simulink model "PassCarModel_RL_config"  (R2024b)
settings: Solver=FixedStepAuto  StartTime=0.0  StopTime=Tf  FixedStep=.001  RelTol=1e-2
StartFcn:
  | %tic
StopFcn:
  | %toc
model workspace (MAT data in the model file):
  AverageTimeInterval = 0.5
  Downshift_Speeds = [9.5625  23.0625  36.5625  47.8125  59.0625  68.90625  78.75; 12.9375  26.4375  39.9375  51.1875  62.4375  72.84375  83.25; 16.3125  29.8125  43.3125  54.5625  65.8125  76.78125  87.75; 19.6875  33.1875  46.6875  57.9375  69.1875  80.71875  92.25]
  EEC_Counter = Simulink.Parameter
  EEC_Counter.Value = 0
  EEC_Counter.Complexity = 'real'
  EEC_Counter.Dimensions = [1 1]
  EEC_Counter.DataType = 'uint8'
  EngRevLim = 7000
  FuzzOffset = Simulink.Parameter
  FuzzOffset.Value = 0
  FuzzOffset.Complexity = 'real'
  FuzzOffset.Dimensions = [1 1]
  FuzzOffset.DataType = 'auto'
  FuzzRange = Simulink.Parameter
  FuzzRange.Value = 60
  FuzzRange.Complexity = 'real'
  FuzzRange.Dimensions = [1 1]
  FuzzRange.DataType = 'auto'
  Fuzzing = Simulink.Parameter
  Fuzzing.Value = 0
  Fuzzing.Complexity = 'real'
  Fuzzing.Dimensions = [1 1]
  Fuzzing.DataType = 'auto'
  Pedal_Positions = [0.1 0.4 0.5 0.9]
  TrackPoints = [0 36.336 72.672 109.008 145.344 181.68 218.016 254.352 290.688 327.024 363.36 403.196036522 ... (360 elements, 120x3)]
  Upshift_Speeds = [12.9375  26.4375  39.9375  51.1875  62.4375  72.84375  83.25; 16.3125  29.8125  43.3125  54.5625  65.8125  76.78125  87.75; 19.6875  33.1875  46.6875  57.9375  69.1875  80.71875  92.25; 33  52.5  77.25  100.5  138.75  161.875  185]
  VEH.Mass = 1181
  VEH.StaticNormalFrontLoad.FR = 264.666666667
  VEH.StaticNormalFrontLoad.FL = 264.666666667
  VEH.StaticNormalRearLoad.RR = 322
  VEH.StaticNormalRearLoad.RL = 322
  VEH.WheelBase = 3.075
  VEH.FrontAxlePositionfromCG = 1.515
  VEH.RearAxlePositionfromCG = 1.504
  VEH.HeightCG = 0.134
  VEH.FrontalArea = 2.11
  VEH.DragCoefficient = 0.33
  VEH.NumberOfWheelsPerAxle = 2
  VEH.PitchMomentInertia = 1922.66666667
  VEH.RollMomentInertia = 432.333333333
  VEH.YawMomentInertia = 2066
  VEH.SteeringRatio = 18
  VEH.TrackWidth = 1.922
  VEH.SprungMass = 1096.72266667
  VEH.InitialLongPosition = 7.25329912144
  VEH.InitialLatPosition = 1.0710379423
  VEH.InitialVertPosition = 0
  VEH.InitialRollAngle = 0
  VEH.InitialPitchAngle = 0
  VEH.InitialYawAngle = 2.62319668541
  VEH.InitialLongVel = 0
  VEH.InitialLatVel = 0
  VEH.InitialVertVel = 0
  VEH.InitialRollRate = 0
  VEH.InitialPitchRate = 0
  VEH.InitialYawRate = 0
  VEH.UnsprungMassRearAxle = 160
  VEH.UnsprungMassFrontAxle = 100
  gradbp = Simulink.Parameter
  gradbp.Value = [0 3.12151852564 6.24303705128 9.36455557691 12.4860741026 15.6075926282 18.7291111538 21.8506296795 24.9721482051 28.0936667307 31.2151852564 34.336703782 37.4582223077 40.5797408333 43.7012593589 46.8227778846 49.9442964102 53.0658149359 56.1873334615 59.3088519871 62.4303705128 65.5518890384 68.673407564 71.7949260897 74.9164446153 78.037963141 81.1594816666 84.2810001922 87.4025187179 90.5240372435 93.6455557691 96.7670742948 99.8885928204 103.010111346 106.131629872 109.253148397 112.374666923 115.496185449 118.617703974 121.7392225]
  gradbp.Complexity = 'real'
  gradbp.Dimensions = [1 40]
  gradbp.DataType = 'auto'
  origin = Simulink.Parameter
  origin.Value = [47.47664 19.05601 0]
  origin.Complexity = 'real'
  origin.Dimensions = [1 3]
  origin.DataType = 'auto'
  rayDirections = [0  0  -1; 0  0  -1; 0  0  -1; 0  0  -1; 0  0  -1; 0  0  -1; 0  0  -1; 0  0  -1; 0  0  -1; 0  0  -1; 0  0  -1; 0  0  -1; 0  0  -1; 0  0  -1; 0  0  -1; 0  0  -1; 0  0  -1; 0  0  -1; 0  0  -1; 0  0  -1; 0  0  -1; 0  0  -1; 0  0  -1; 0  0  -1; 0  0  -1; 0  0  -1; 0  0  -1; 0  0  -1; 0  0  -1; 0  0  -1; 0  0  -1; 0  0  -1; 0  0  -1; 0  0  -1; 0  0  -1; 0  0  -1; 0  0  -1; 0  0  -1; 0  0  -1; 0  0  -1; 0  0  -1; 0  0  -1; 0  0  -1; 0  0  -1; 0  0  -1; 0  0  -1; 0  0  -1; 0  0  -1; 0  0  -1; 0  0  -1; 0  0  -1; 0  0  -1; 0  0  -1; 0  0  -1; 0  0  -1; 0  0  -1; 0  0  -1; 0  0  -1; 0  0  -1; 0  0  -1; 0  0  -1; 0  0  -1; 0  0  -1; 0  0  -1; 0  0  -1; 0  0  -1; 0  0  -1; 0  0  -1; 0  0  -1; 0  0  -1; 0  0  -1; 0  0  -1; 0  0  -1; 0  0  -1; 0  0  -1; 0  0  -1; 0  0  -1; 0  0  -1; 0  0  -1; 0  0  -1; 0  0  -1; 0  0  -1; 0  0  -1; 0  0  -1; 0  0  -1; 0  0  -1; 0  0  -1; 0  0  -1; 0  0  -1; 0  0  -1; 0  0  -1; 0  0  -1; 0  0  -1; 0  0  -1; 0  0  -1; 0  0  -1; 0  0  -1; 0  0  -1; 0  0  -1; 0  0  -1; 0  0  -1; 0  0  -1; 0  0  -1; 0  0  -1; 0  0  -1; 0  0  -1; 0  0  -1; 0  0  -1; 0  0  -1; 0  0  -1; 0  0  -1; 0  0  -1; 0  0  -1; 0  0  -1; 0  0  -1; 0  0  -1; 0  0  -1; 0  0  -1; 0  0  -1; 0  0  -1; 0  0  -1]
  rayLengths = [20; 20; 20; 20; 20; 20; 20; 20; 20; 20; 20; 20; 20; 20; 20; 20; 20; 20; 20; 20; 20; 20; 20; 20; 20; 20; 20; 20; 20; 20; 20; 20; 20; 20; 20; 20; 20; 20; 20; 20; 20; 20; 20; 20; 20; 20; 20; 20; 20; 20; 20; 20; 20; 20; 20; 20; 20; 20; 20; 20; 20; 20; 20; 20; 20; 20; 20; 20; 20; 20; 20; 20; 20; 20; 20; 20; 20; 20; 20; 20; 20; 20; 20; 20; 20; 20; 20; 20; 20; 20; 20; 20; 20; 20; 20; 20; 20; 20; 20; 20; 20; 20; 20; 20; 20; 20; 20; 20; 20; 20; 20; 20; 20; 20; 20; 20; 20; 20; 20; 20; 20]
  rayOrigins = [0.5  -0.5  0; 0.4  -0.5  0; 0.3  -0.5  0; 0.2  -0.5  0; 0.1  -0.5  0; 0  -0.5  0; -0.1  -0.5  0; -0.2  -0.5  0; -0.3  -0.5  0; -0.4  -0.5  0; -0.5  -0.5  0; 0.5  -0.4  0; 0.4  -0.4  0; 0.3  -0.4  0; 0.2  -0.4  0; 0.1  -0.4  0; 0  -0.4  0; -0.1  -0.4  0; -0.2  -0.4  0; -0.3  -0.4  0; -0.4  -0.4  0; -0.5  -0.4  0; 0.5  -0.3  0; 0.4  -0.3  0; 0.3  -0.3  0; 0.2  -0.3  0; 0.1  -0.3  0; 0  -0.3  0; -0.1  -0.3  0; -0.2  -0.3  0; -0.3  -0.3  0; -0.4  -0.3  0; -0.5  -0.3  0; 0.5  -0.2  0; 0.4  -0.2  0; 0.3  -0.2  0; 0.2  -0.2  0; 0.1  -0.2  0; 0  -0.2  0; -0.1  -0.2  0; -0.2  -0.2  0; -0.3  -0.2  0; -0.4  -0.2  0; -0.5  -0.2  0; 0.5  -0.1  0; 0.4  -0.1  0; 0.3  -0.1  0; 0.2  -0.1  0; 0.1  -0.1  0; 0  -0.1  0; -0.1  -0.1  0; -0.2  -0.1  0; -0.3  -0.1  0; -0.4  -0.1  0; -0.5  -0.1  0; 0.5  0  0; 0.4  0  0; 0.3  0  0; 0.2  0  0; 0.1  0  0; 0  0  0; -0.1  0  0; -0.2  0  0; -0.3  0  0; -0.4  0  0; -0.5  0  0; 0.5  0.1  0; 0.4  0.1  0; 0.3  0.1  0; 0.2  0.1  0; 0.1  0.1  0; 0  0.1  0; -0.1  0.1  0; -0.2  0.1  0; -0.3  0.1  0; -0.4  0.1  0; -0.5  0.1  0; 0.5  0.2  0; 0.4  0.2  0; 0.3  0.2  0; 0.2  0.2  0; 0.1  0.2  0; 0  0.2  0; -0.1  0.2  0; -0.2  0.2  0; -0.3  0.2  0; -0.4  0.2  0; -0.5  0.2  0; 0.5  0.3  0; 0.4  0.3  0; 0.3  0.3  0; 0.2  0.3  0; 0.1  0.3  0; 0  0.3  0; -0.1  0.3  0; -0.2  0.3  0; -0.3  0.3  0; -0.4  0.3  0; -0.5  0.3  0; 0.5  0.4  0; 0.4  0.4  0; 0.3  0.4  0; 0.2  0.4  0; 0.1  0.4  0; 0  0.4  0; -0.1  0.4  0; -0.2  0.4  0; -0.3  0.4  0; -0.4  0.4  0; -0.5  0.4  0; 0.5  0.5  0; 0.4  0.5  0; 0.3  0.5  0; 0.2  0.5  0; 0.1  0.5  0; 0  0.5  0; -0.1  0.5  0; -0.2  0.5  0; -0.3  0.5  0; -0.4  0.5  0; -0.5  0.5  0]
  theta = Simulink.Parameter
  theta.Value = [0.635451508064; 0.635451508064; 0.635451508064; 0.635451508064; 0.635451508064; 0.635451508064; 0.635451508064; 0.624762119358; 0.623142229392; 0.621522339426; 0.619902449459; 0.618282559493; 0.616662669527; 0.615042779561; 0.613422889595; 0.611802999629; 0.611153158573; 0.611153158573; 0.611153158573; 0.611153158573; 0.611153158573; 0.611153158573; 0.611153158573; 0.611153158573; 0.611278748463; 0.622335874545; 0.621279829225; 0.620168434025; 0.619057038825; 0.617945643626; 0.616834248426; 0.615722853226; 0.614611458026; 0.595312478773; 0.594482230575; 0.594482230575; 0.594482230575; 0.594482230575; 0.594482230575; 0.594482230575]
  theta.Complexity = 'real'
  theta.Dimensions = [40 1]
  theta.DataType = 'auto'
  totalDistance = Simulink.Parameter
  totalDistance.Value = 121.7392225
  totalDistance.Complexity = 'real'
  totalDistance.Dimensions = [1 1]
  totalDistance.DataType = 'auto'
  vel_profile3 = Simulink.Parameter
  vel_profile3.Value = [1; 4.4417464081; 5.58369016682; 7.3294091164; 8.57061065054; 9.62904493054; 10.5728796274; 11.4345982514; 12.2332634698; 12.981352122; 13.6876153753; 14.358495835; 14.9989108849; 15.5865267169; 16.0408872489; 16.3678958423; 16.5727345417; 16.66; 16.66; 16.66; 16.66; 16.66; 16.66; 16.66; 16.66; 16.66; 16.66; 16.66; 16.66; 16.66; 16.66; 16.66; 16.66; 16.66; 16.66; 15.8266070222; 12.4946070222; 9.16260702218; 0; 0]
  vel_profile3.Complexity = 'real'
  vel_profile3.Dimensions = [40 1]
  vel_profile3.DataType = 'auto'
  xEast = Simulink.Parameter
  xEast.Value = [0; 2.51220993996; 5.02441987992; 7.53662981988; 10.0488397598; 12.5610496998; 15.0732596398; 17.5854695797; 20.0976795197; 22.6364013732; 25.1928840476; 27.7493667221; 30.3058493965; 32.862332071; 35.4188147455; 37.9752974199; 40.5317800944; 43.0882627688; 45.6447454433; 48.2012281178; 50.7577107922; 53.3141934667; 55.8706761411; 58.4271588156; 60.9836414901; 63.5401241645; 66.096606839; 68.6530895134; 71.2095721879; 73.7660548624; 76.3225375368; 78.8790202113; 81.4317288843; 83.6574125711; 86.2417511267; 88.8277375705; 91.4137240144; 93.9997104582; 96.5856969021; 99.1716833459]
  xEast.Complexity = 'real'
  xEast.Dimensions = [40 1]
  xEast.DataType = 'auto'
  yNorth = Simulink.Parameter
  yNorth.Value = [0; 1.85274907191; 3.70549814382; 5.55824721574; 7.41099628765; 9.26374535956; 11.1164944315; 12.9692435034; 14.8219925753; 16.6378635224; 18.429029132; 20.2201947417; 22.0113603513; 23.8025259609; 25.5936915705; 27.3848571802; 29.1760227898; 30.9671883994; 32.758354009; 34.5495196186; 36.3406852283; 38.1318508379; 39.9230164475; 41.7141820571; 43.5053476667; 45.2965132764; 47.087678886; 48.8788444956; 50.6700101052; 52.4611757148; 54.2523413245; 56.0435069341; 57.8392073973; 60.0278622426; 61.7781760106; 63.5264757613; 65.2747755119; 67.0230752625; 68.7713750132; 70.5196747638]
  yNorth.Complexity = 'real'
  yNorth.Dimensions = [40 1]
  yNorth.DataType = 'auto'
undefined symbols (not defined in the file or in its folder): DecelR, DiscIntNeverNeededParam, dspblkCoreblockFVToolHelper, FO_max, FO_min, FR_max, FR_min, gcbh, ODevR, Sim3dSensor, Ts
libraries: simulink x20, dspstat3 x8, autolibutils x6, sim3dgroundtruthsensorlib x2, rllib x1, slpidlib x1, autolibtranscontrolscommon x1, vehdynlibdriver x1, sharedtransform x1, vehdynlibviscommon x1, vehdynlibsens x1
(part 1 of 5)
settings Model: DataDictionary=VehicleConfig.sldd  SimulationMode=accelerator  PauseTimes=23.4  PacingRate=0.400000  Creator=The MathWorks, Inc.  LastModifiedBy=user
settings SolverCC: SolverJacobianMethodControl=FullPerturbation  ZeroCrossAlgorithm=Adaptive  AlgebraicLoopSolver=TrustRegion  AutoInsertRateTranBlk=on  InsertRTBMode=Never (minimum delay)  DecoupledContinuousIntegration=on  MinimalZcImpactIntegration=on  MaxZcPerStep=1
settings DataIOCC: DSMLogging=off
settings OptimizationCC: UseDivisionForNetSlopeComputation=on  UseFloatMulNetSlope=on  OptimizeBlockIOStorage=off  BufferReuse=off  ReuseModelBlockBuffer=off  GlobalBufferReuse=off  ExpressionFolding=off  EnableMemcpy=off  PassReuseOutputArgsAs=Individual arguments  LocalBlockOutputs=off  ZeroExternalMemoryAtStartup=off  ZeroInternalMemoryAtStartup=off  EfficientFloat2IntCast=on  OptimizeDataStoreBuffers=off  BusAssignmentInplaceUpdate=off  OptimizationLevel=level0  OptimizationCustomize=off  EfficientTunableParamExpr=on
settings DebuggingCC: ReadBeforeWriteMsg=DisableAll  WriteAfterWriteMsg=DisableAll  WriteAfterReadMsg=DisableAll  ArtificialAlgebraicLoopMsg=none  MaskedZcDiagnostic=none  IgnoredZcDiagnostic=none  InheritedTsInSrcMsg=none  MultiTaskDSMMsg=none  IntegerOverflowMsg=none  ParamPrecisionLossAbsoluteDiffThreshold=1e-06  ParameterTunabilityLossMsg=error  UnconnectedInputMsg=warning  UnconnectedOutputMsg=warning  UnconnectedLineMsg=warning  PregeneratedLibrarySubsystemCodeDiagnostic=none  ArithmeticOperatorsInVariantConditions=warning
settings HardwareCC: ProdLongLongMode=on  TargetBitPerPointer=64  TargetBitPerSizeT=64  TargetBitPerPtrDiffT=64  TargetLongLongMode=on  TargetIntDivRoundTo=Zero  TargetEndianess=LittleEndian  TargetWordSize=64  TargetHWDeviceType=MATLAB Host  ProdEqTarget=off
settings ModelReferenceCC: UpdateModelReferenceTargets=IfOutOfDate  EnableRefExpFcnMdlSchedulingChecks=on  ModelReferenceMinAlgLoopOccurrences=on  PropagateSignalLabelsOutOfModel=off
settings SFSimCC: SimUseLocalCustomCode=off  MATLABDynamicMemAlloc=off
settings RTWCC: Description=Embedded Coder (host-based shared library target)  SystemTargetFile=ert_shrlib.tlc  TemplateMakefile=ert_default_tmf  PostCodeGenCommand=packNGo(buildInfo)  RTWUseLocalCustomCode=off  GPUComputeCapability=3.5  DLArmComputeVersion=19.05
settings CodeAppCC: ForceParamTrailComments=on  IgnoreCustomStorageClasses=off  MaxIdLength=50  OperatorAnnotations=on  SimulinkDataObjDesc=on  SFDataObjDesc=on  InsertBlockDesc=on
settings STFCustomTargetCC: TargetLangStandard=C99 (ISO)  MultiwordLength=256  GenerateSampleERTMain=on  ParMdlRefBuildCompliant=on  CompOptLevelCompliant=on  CombineOutputUpdateFcns=on  ERTCustomFileBanners=on  SupportNonInlinedSFcns=off  RemoveResetFunc=on  SupportVariableSizeSignals=on  MATLABClassNameForMDSCustomization=Simulink.SoftwareTarget.ERTCustomization  ModelStepFunctionPrototypeControlCompliant=on  UseToolchainInfoCompliant=on  SystemTargetFile=ert_shrlib.tlc
settings ERTTargetCC: TargetLangStandard=C99 (ISO)  GenerateSampleERTMain=on  ConcurrentExecutionCompliant=off  SupportContinuousTime=on  SupportVariableSizeSignals=on  CPPClassGenCompliant=off  InlinedParameterPlacement=Hierarchical  ERTCustomFileTemplate=example_file_process.tlc

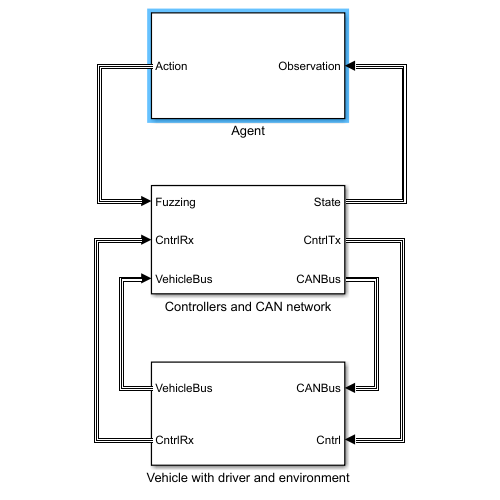
[thumbnail: Simulink's stored preview of the top-level diagram]
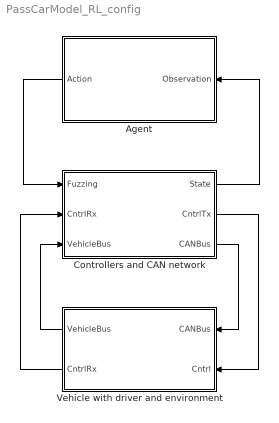
== system PassCarModel_RL_config ==
  Agent : Subsystem
  Controllers and CAN network : Subsystem
  Vehicle with driver and environment : Subsystem
  wires:
  Vehicle with driver and environment/1(VehicleBus) -> Controllers and CAN network/3(VehicleBus)
  Vehicle with driver and environment/2(CntrlRx) -> Controllers and CAN network/2(CntrlRx)
  Controllers and CAN network/2(CntrlTx) -> Vehicle with driver and environment/2(Cntrl)
  Controllers and CAN network/3(CANBus) -> Vehicle with driver and environment/1(CANBus)
  Controllers and CAN network/1(State) -> Agent/1(Observation)
  Agent/1(Action) -> Controllers and CAN network/1(Fuzzing)

== system PassCarModel_RL_config/Agent ==
  Observation : Inport
  Abs : Abs  SaturateOnIntegerOverflow=off
  Abs1 : Abs  SaturateOnIntegerOverflow=off
  Abs2 : Abs  SaturateOnIntegerOverflow=off
  Add : Sum  Inputs=+++
  Bus Selector : BusSelector  OutputSignals=AvgVehSpeed,AvgOmega
  Bus Selector1 : BusSelector  OutputSignals=AvgDecel,AvgLatAcc,OmegaDeviation
  Bus Selector2 : BusSelector  OutputSignals=AvgVehSpeed
  DecelR : Gain  Gain=DecelR
  Gain : Gain  Gain=-Ts/0.1
  Mux : Mux  Inputs=2
  ODevR : Gain  Gain=ODevR
  Policy : Subsystem
  RL Agent : rllib/RL Agent  Agent=agent  ExternalActionAsInput=off  ProvideLastAction=off  ProvideCumRwd=off  TreatAsDirectFeedthrough=on  UseStrictObservationDataTypes=off
  Relational Operator : RelationalOperator  Operator=<=  OutDataTypeStr=boolean  RndMeth=Simplest  InputSameDT=off
  StoppingCondition : Constant  Value=0.1
  Action : Outport
  wires:
  Relational Operator/1 -> RL Agent/3
  Gain/1 -> RL Agent/2  "Reward"
  Bus Selector1/3 -> Abs2/1  "<OmegaDeviation>"
  Bus Selector1/1 -> Abs/1  "<AvgDecel>"
  StoppingCondition/1 -> Relational Operator/2
  Abs1/1 -> Add/2
  RL Agent/1 -> Policy/1(action)
  Bus Selector1/2 -> Abs1/1  "<AvgLatAcc>"
  Bus Selector/1 -> Mux/1  "<AvgVehSpeed>"
  Abs/1 -> DecelR/1
  Observation/1 -> Bus Selector2/1, Bus Selector/1, Bus Selector1/1
  Add/1 -> Gain/1
  Mux/1 -> RL Agent/1  "Observation"
  Bus Selector2/1 -> Relational Operator/1  "<AvgVehSpeed>"
  Bus Selector/2 -> Mux/2  "<AvgOmega>"
  Policy/1(Action) -> Action/1  "FuzzingAction"
  Abs2/1 -> ODevR/1
  DecelR/1 -> Add/1
  ODevR/1 -> Add/3

== system PassCarModel_RL_config/Controllers and CAN network ==
  Fuzzing : Inport
  CntrlRx : Inport  Port=2
  VehicleBus : Inport  Port=3
  CAN : Subsystem
  Controllers : Subsystem
      mask Display: image('SystemControllers.png')
  Gateway : Subsystem
  Monitoring : Subsystem
  State : Outport
  CntrlTx : Outport  Port=2
  CANBus : Outport  Port=3
  wires:
  Gateway/1(OmegaFuzz) -> Monitoring/2(OmegaFuzz)
  VehicleBus/1 -> CAN/1(VehFdbk), Gateway/1(VehicleBus), Monitoring/1(VehicleBus)
  Gateway/2(CANBusOut) -> Monitoring/3(CANBus), CANBus/1, Controllers/1(CANBus)  "CANBus"
  CAN/1(CANBus) -> Gateway/2(CANBusIn)
  CntrlRx/1 -> Controllers/2(CntrlRx)
  Fuzzing/1 -> CAN/2(Fuzzing)
  Controllers/1(CntrlTx) -> CntrlTx/1
  Monitoring/1(State) -> State/1  "RLState"

== system PassCarModel_RL_config/Vehicle with driver and environment ==
  CANBus : Inport
  Cntrl : Inport  Port=2
  Driver : Subsystem
  Environment : Subsystem
      mask Display: disp('Environment')
  Passenger Vehicle : Subsystem
      mask Display: image('PassengerVehicle.png')
  Sensors : Subsystem
      mask Display: image('sensorimu.png'); % Use "Edit Image" on toolstrip to change.
  VehicleBus : Outport
  CntrlRx : Outport  Port=2
  wires:
  Environment/1(Env) -> Passenger Vehicle/4(Env), Sensors/2(Env)
  Sensors/1(CntrlRx) -> CntrlRx/1
  Passenger Vehicle/1(VehFdbk) -> Driver/1(In1), VehicleBus/1, Environment/1(VehFdbk), Sensors/1(VehFdbk)  "VehicleBus"
  Driver/1(Out1) -> Passenger Vehicle/1(Driver)
  Cntrl/1 -> Passenger Vehicle/2(Cntrl)
  CANBus/1 -> Passenger Vehicle/3(CANBus)

== system PassCarModel_RL_config/Agent/Policy ==
  action : Inport
  Bus Creator : BusCreator  Inputs=4
  Constant : Constant  Value=(FO_max+FO_min)/2
  Constant1 : Constant  Value=(FO_max-FO_min)/2
  Constant2 : Constant  Value=(FR_max+FR_min)/2
  Constant3 : Constant  Value=(FR_max-FR_min)/2
  Demux : Demux  Outputs=2
  Fuzzing : Constant
  MATLAB Function : MATLAB Function  TreatAsAtomicUnit=on
  Product : Product
  Product1 : Product
  Sum : Sum  Inputs=|++
  Sum1 : Sum  Inputs=|++
  UniformNormal : Constant  Value=0
  Action : Outport
  wires:
  Bus Creator/1 -> Action/1  "Action"
  Sum1/1 -> Bus Creator/4  "FuzzingRange"
  Fuzzing/1 -> Bus Creator/1  "Fuzzing"
  UniformNormal/1 -> Bus Creator/2  "UniformNormal"
  Sum/1 -> Bus Creator/3  "FuzzingOffset"
  Demux/1 -> Product/2
  Constant1/1 -> Product/1
  Constant/1 -> Sum/2
  Product/1 -> Sum/1
  Product1/1 -> Sum1/1
  Constant2/1 -> Sum1/2
  Constant3/1 -> Product1/1
  Demux/2 -> Product1/2
  action/1 -> MATLAB Function/1(u)
  MATLAB Function/1(y) -> Demux/1

== system PassCarModel_RL_config/Controllers and CAN network/CAN ==
  VehFdbk : Inport
  Fuzzing : Inport  Port=2
  BrakeController : Subsystem
  Bus Creator : BusCreator  Inputs=4
  CentralController : Subsystem
  EngineController : Subsystem
  TransmissionController : Subsystem
  CANBus : Outport
  wires:
  VehFdbk/1 -> TransmissionController/1(VehDataBus), CentralController/1(VehDataBus), BrakeController/2(VehDataBus), EngineController/1(VehDataBus)  "VehDataBus"
  BrakeController/1(BrakeController) -> Bus Creator/1  "BrakeController"
  EngineController/1(EngineController) -> Bus Creator/2  "EngineController"
  TransmissionController/1(TransmissionController) -> Bus Creator/3  "TransmissionController"
  CentralController/1(CentralController) -> Bus Creator/4  "CentralController"
  Bus Creator/1 -> CANBus/1
  Fuzzing/1 -> BrakeController/1(Fuzzing)

== system PassCarModel_RL_config/Controllers and CAN network/Controllers ==
  CANBus : Inport
  CntrlRx : Inport  Port=2
  ADCMode : Subsystem
  Active Differential Control : Subsystem  Variant=on  VariantControlMode=label  LabelModeActiveChoice=0
  BCMode : Subsystem  mask{ControlMode=CAN}
      mask prompts: ControlMode "Select control mode"
      mask DialogControl DescTextVar Prompt: If CAN is selected the control signals are received from the CAN bus.
  Brake Pressure Control : Subsystem  Variant=on  VariantControlMode=label  LabelModeActiveChoice=Slip control
  Bus Creator : BusCreator  Inputs=1
  Bus Creator1 : BusCreator  Inputs=1
  Bus Creator2 : BusCreator  Inputs=3
  Bus Creator3 : BusCreator  Inputs=4
  Bus Creator4 : BusCreator  Inputs=1
  ECMode : Subsystem  mask{ControlMode=CAN}
      mask prompts: ControlMode "Select control mode"
      mask DialogControl DescTextVar Prompt: If CAN is selected the control signals are received from the CAN bus.
  ECU : Subsystem  SystemSampleTime=.01
  Ground : Ground
  Logical Operator : Logic  Operator=OR  Inputs=1  AllPortsSameDT=off  OutDataTypeStr=boolean
  TCMode : Subsystem  mask{ControlMode=CAN}
      mask prompts: ControlMode "Select control mode"
      mask DialogControl DescTextVar Prompt: If CAN is selected the control signals are received from the CAN bus.
  Terminator : Terminator
  Transmission Controller : Subsystem  Variant=on  VariantControlMode=label  VariantControl=Variant1  LabelModeActiveChoice=3
  CntrlTx : Outport  VectorParamsAs1DForOutWhenUnconnected=off
  wires:
  Bus Creator/1 -> Bus Creator3/1  "ECU"
  Bus Creator1/1 -> Bus Creator3/2  "Transmission"
  Bus Creator3/1 -> CntrlTx/1  "CntrlTx"
  Bus Creator4/1 -> Bus Creator3/4  "Diff"
  Active Differential Control/1(DiffPrsCmd) -> Bus Creator4/1  "DiffPrsCmd"
  Active Differential Control/2(TrqCmd) -> [DiffTrqCmd]
  ECU/1(EngTrqCmd) -> Bus Creator/1  "EngTrqCmd"
  Transmission Controller/1(" Gear") -> Bus Creator1/1  "GearCmd"
  [DiffTrqCmd] -> ECU/1(DiffTrqCmd)  "DiffTrqCmd"
  Ground/1 -> Transmission Controller/7(UpReq), Transmission Controller/8(DownReq)
  Brake Pressure Control/2(BrkPrsCmd) -> Bus Creator2/2  "BrkPrsCmd"
  Bus Creator2/1 -> Bus Creator3/3  "Brake"
  Brake Pressure Control/1(ABSFlag) -> [ABSFlag], Logical Operator/1, Bus Creator2/1  "ABSFlag"
  ECMode/3(<ABSFlag>) -> ECU/4(ABSFlag)
  Brake Pressure Control/3(TCSFlag) -> Bus Creator2/3  "TCSFlag"
  TCMode/1(<AccFdbk>) -> Transmission Controller/1(Accel)
  TCMode/2(<DecelFdbk>) -> Transmission Controller/2(BrkCmd)
  TCMode/3(<GearFdbk>) -> Transmission Controller/3(GearReq)
  TCMode/4(<EngSpd>) -> Transmission Controller/4(EngSpd)
  TCMode/5(<Omega>) -> Transmission Controller/5(Omega)
  BCMode/1(<DecelFdbk>) -> Brake Pressure Control/1(DecelFdbk)
  BCMode/2(<Omega>) -> Brake Pressure Control/2(Omega)
  BCMode/3(Accel) -> Brake Pressure Control/3(Accel)
  BCMode/4(<AccFdbk>) -> Brake Pressure Control/4(AccelFdbk)
  BCMode/5(<BrkPrs>) -> Brake Pressure Control/5(BrkPrs)
  [ABSFlag] -> ECMode/3(ABSFlag)
  ECMode/1(<AccFdbk>) -> ECU/2(<Accel>)
  ECMode/2(<EngSpd>) -> ECU/3(EngSpd)
  [ABSFlag] -> TCMode/3(ABSFlag)
  TCMode/6(<ABSFlag>) -> Transmission Controller/6(ABSFlag)
  ADCMode/1(<AccFdbk>) -> Active Differential Control/1(Accel)
  ADCMode/2(<DecelFdbk>) -> Active Differential Control/2(BrkCmd)
  ADCMode/3(<SteerFdbk>) -> Active Differential Control/3(Steer)
  ADCMode/4(<GearFdbk>) -> Active Differential Control/4(GearFdbk)
  ADCMode/5(<Omega>) -> Active Differential Control/5(Omega)
  ADCMode/6(<Acc>) -> Active Differential Control/6(axayaz)
  ADCMode/7(<pqr>) -> Active Differential Control/7(pqr)
  Logical Operator/1 -> Terminator/1  "ABS_active"
  CANBus/1 -> BCMode/2(CANBus), TCMode/2(CANBus), ECMode/2(CANBus)
  CntrlRx/1 -> ECMode/1(CntrlRx), TCMode/1(CntrlRx), BCMode/1(CntrlRx), ADCMode/1(In1)

== system PassCarModel_RL_config/Controllers and CAN network/Gateway ==
  VehicleBus : Inport
  CANBusIn : Inport  Port=2
  BC-Filter : Subsystem
  Bus Creator : BusCreator  Inputs=4
  Bus Selector : BusSelector  OutputSignals=EngineController,BrakeController,CentralController,TransmissionController
  Terminator : Terminator
  OmegaFuzz : Outport
  CANBusOut : Outport  Port=2
  wires:
  Bus Creator/1 -> CANBusOut/1
  Bus Selector/4 -> [TC]  "<TransmissionController>"
  Bus Selector/3 -> [CC]  "<CentralController>"
  Bus Selector/2 -> Terminator/1  "<BrakeController>"
  Bus Selector/1 -> [EC]  "<EngineController>"
  CANBusIn/1 -> BC-Filter/2(CANBus), Bus Selector/1
  [EC] -> Bus Creator/1
  BC-Filter/1(BrakeController) -> Bus Creator/2  "BrakeController"
  [CC] -> Bus Creator/3
  [TC] -> Bus Creator/4
  VehicleBus/1 -> BC-Filter/1(VehicleBus)
  BC-Filter/2(OmegaFuzz) -> OmegaFuzz/1

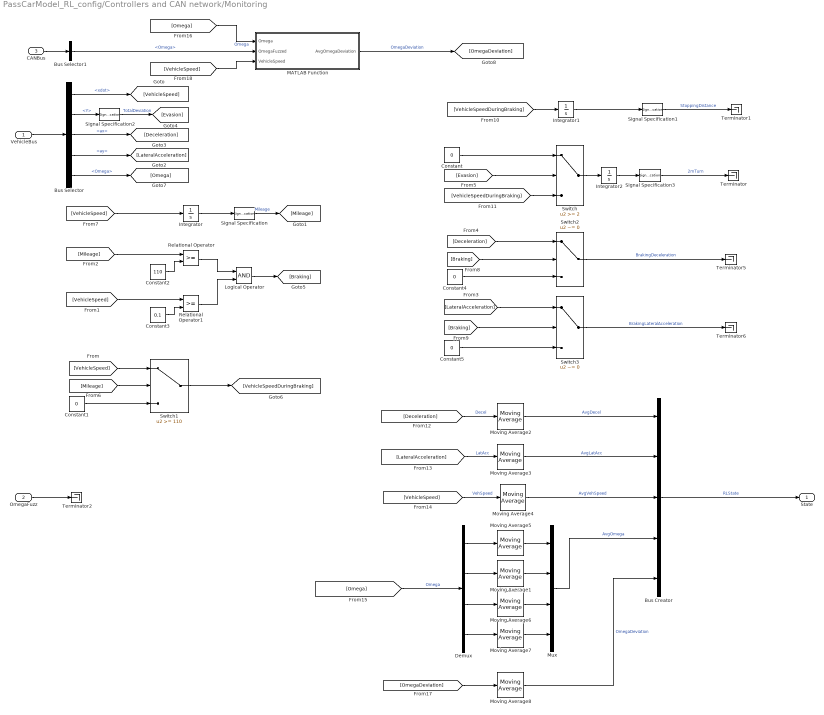
== system PassCarModel_RL_config/Controllers and CAN network/Monitoring ==
  VehicleBus : Inport
  OmegaFuzz : Inport  Port=2
  CANBus : Inport  Port=3
  Bus Creator : BusCreator  Inputs=5
  Bus Selector : BusSelector  OutputSignals=Body.BdyFrm.Cg.Vel.xdot,Body.InertFrm.Cg.Disp.Y,Body.BdyFrm.Cg.Acc.ax,Body.BdyFrm.Cg.Acc.ay,Wheels.TireFrame.Omega
  Bus Selector1 : BusSelector  OutputSignals=BrakeController.Omega
  Constant{,1,4..5} (4 alike) : Constant  Value=0
  Constant2 : Constant  Value=110
  Constant3 : Constant  Value=0.1
  Demux : Demux
  Integrator : Integrator
  Integrator1 : Integrator
  Integrator2 : Integrator
  Logical Operator : Logic  AllPortsSameDT=off  OutDataTypeStr=boolean
  MATLAB Function : MATLAB Function  TreatAsAtomicUnit=on
  Moving Average{1,5..8} (5 alike) : dspstat3/Moving Average  Method=Sliding window  ForgettingFactorPort=off  SpecifyWindowLength=on  WindowLength=50  OverlapLength=49  AllowArbitraryInputLength=off  ForgettingFactor=0.9  SimulateUsing=Code generation
  Moving Average2 : dspstat3/Moving Average  Method=Sliding window  ForgettingFactorPort=off  SpecifyWindowLength=on  WindowLength=500  OverlapLength=499  AllowArbitraryInputLength=off  ForgettingFactor=0.9  SimulateUsing=Code generation
  Moving Average3 : dspstat3/Moving Average  Method=Sliding window  ForgettingFactorPort=off  SpecifyWindowLength=on  WindowLength=500  OverlapLength=499  AllowArbitraryInputLength=off  ForgettingFactor=0.9  SimulateUsing=Code generation
  Moving Average4 : dspstat3/Moving Average  Method=Sliding window  ForgettingFactorPort=off  SpecifyWindowLength=on  WindowLength=500  OverlapLength=499  AllowArbitraryInputLength=off  ForgettingFactor=0.9  SimulateUsing=Code generation
  Mux : Mux
  Relational Operator : RelationalOperator  OutDataTypeStr=boolean  RndMeth=Simplest  InputSameDT=off
  Relational Operator1 : RelationalOperator  OutDataTypeStr=boolean  RndMeth=Simplest  InputSameDT=off
  Signal Specification{,1..3} (4 alike) : SignalSpecification  Unit=m
  Switch : Switch  Threshold=2  SaturateOnIntegerOverflow=off  InputSameDT=off
  Switch1 : Switch  Threshold=110  SaturateOnIntegerOverflow=off  InputSameDT=off
  Switch2 : Switch  Criteria=u2 ~= 0  SaturateOnIntegerOverflow=off  InputSameDT=off
  Switch3 : Switch  Criteria=u2 ~= 0  SaturateOnIntegerOverflow=off  InputSameDT=off
  Terminator{,1..2,5..6} (5 alike) : Terminator
  State : Outport
  wires:
  [VehicleSpeed] -> Switch1/1
  Integrator/1 -> Signal Specification/1
  Signal Specification/1 -> [Mileage]  "Mileage"
  VehicleBus/1 -> Bus Selector/1
  Bus Selector/2 -> Signal Specification2/1  "<Y>"
  Constant/1 -> Switch/1
  Constant1/1 -> Switch1/3
  Integrator1/1 -> Signal Specification1/1
  Switch1/1 -> [VehicleSpeedDuringBraking]
  Signal Specification1/1 -> Terminator1/1  "StoppingDistance"
  Signal Specification2/1 -> [Evasion]  "TotalDeviation"
  CANBus/1 -> Bus Selector1/1
  Switch/1 -> Integrator2/1
  Integrator2/1 -> Signal Specification3/1
  Signal Specification3/1 -> Terminator/1  "2mTurn"
  [Deceleration] -> Switch2/1
  [LateralAcceleration] -> Switch3/1
  Constant2/1 -> Relational Operator/2
  Constant3/1 -> Relational Operator1/2
  Relational Operator/1 -> Logical Operator/1
  Relational Operator1/1 -> Logical Operator/2
  Constant4/1 -> Switch2/3
  Constant5/1 -> Switch3/3
  Switch2/1 -> Terminator5/1  "BrakingDeceleration"
  Switch3/1 -> Terminator6/1  "BrakingLateralAcceleration"
  Bus Selector/1 -> [VehicleSpeed]  "<xdot>"
  [VehicleSpeed] -> Relational Operator1/1
  [Mileage] -> Relational Operator/1
  Bus Selector/4 -> [LateralAcceleration]  "<ay>"
  Bus Selector/3 -> [Deceleration]  "<ax>"
  [Evasion] -> Switch/2
  [Mileage] -> Switch1/2
  [VehicleSpeed] -> Integrator/1
  Logical Operator/1 -> [Braking]
  [Braking] -> Switch2/2
  [Braking] -> Switch3/2
  [VehicleSpeedDuringBraking] -> Integrator1/1
  [VehicleSpeedDuringBraking] -> Switch/3
  [LateralAcceleration] -> Moving Average3/1  "LatAcc"
  Bus Selector/5 -> [Omega]  "<Omega>"
  [Omega] -> Demux/1  "Omega"
  [VehicleSpeed] -> Moving Average4/1  "VehSpeed"
  [Deceleration] -> Moving Average2/1  "Decel"
  Moving Average2/1 -> Bus Creator/1  "AvgDecel"
  Moving Average3/1 -> Bus Creator/2  "AvgLatAcc"
  Moving Average4/1 -> Bus Creator/3  "AvgVehSpeed"
  Moving Average5/1 -> Mux/1
  Bus Creator/1 -> State/1  "RLState"
  Demux/1 -> Moving Average5/1
  Demux/2 -> Moving Average1/1
  Demux/3 -> Moving Average6/1
  Demux/4 -> Moving Average7/1
  Moving Average1/1 -> Mux/2
  Moving Average6/1 -> Mux/3
  Moving Average7/1 -> Mux/4
  Mux/1 -> Bus Creator/4  "AvgOmega"
  [OmegaDeviation] -> Moving Average8/1
  Bus Selector1/1 -> MATLAB Function/2(OmegaFuzzed)  "<Omega>"
  [Omega] -> MATLAB Function/1(Omega)  "Omega"
  [VehicleSpeed] -> MATLAB Function/3(VehicleSpeed)
  MATLAB Function/1(AvgOmegaDeviation) -> [OmegaDeviation]  "OmegaDeviation"
  OmegaFuzz/1 -> Terminator2/1
  Moving Average8/1 -> Bus Creator/5  "OmegaDeviation"

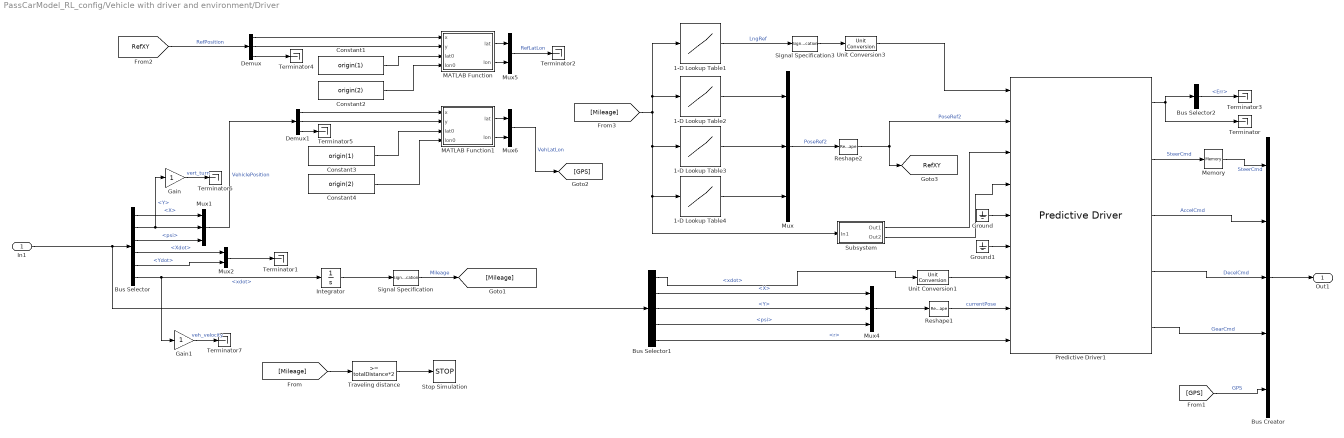
== system PassCarModel_RL_config/Vehicle with driver and environment/Driver ==
  In1 : Inport
  1-D Lookup Table1 : Lookup_n-D  NumberOfTableDimensions=1  BreakpointsForDimension1=gradbp  BeginIndexSearchUsingPreviousIndexResult=on  Table=vel_profile3  ExtrapMethod=Clip  UseLastTableValue=on  InternalRulePriority=Speed  RndMeth=Simplest
  1-D Lookup Table2 : Lookup_n-D  NumberOfTableDimensions=1  BreakpointsForDimension1=gradbp  BeginIndexSearchUsingPreviousIndexResult=on  Table=xEast  ExtrapMethod=Clip  InternalRulePriority=Speed  RndMeth=Simplest
  1-D Lookup Table3 : Lookup_n-D  NumberOfTableDimensions=1  BreakpointsForDimension1=gradbp  BeginIndexSearchUsingPreviousIndexResult=on  Table=yNorth  ExtrapMethod=Clip  InternalRulePriority=Speed  RndMeth=Simplest
  1-D Lookup Table4 : Lookup_n-D  NumberOfTableDimensions=1  BreakpointsForDimension1=gradbp  BeginIndexSearchUsingPreviousIndexResult=on  Table=theta  ExtrapMethod=Clip  InternalRulePriority=Speed  RndMeth=Simplest
  Bus Creator : BusCreator  Inputs=5
  Bus Selector : BusSelector  OutputSignals=Body.InertFrm.Cg.Disp.X,Body.InertFrm.Cg.Disp.Y,Body.InertFrm.Cg.Ang.psi,Body.InertFrm.Cg.Vel.Xdot,Body.InertFrm.Cg.Vel.Ydot,Body.BdyFrm.Cg.Vel.xdot
  Bus Selector1 : BusSelector  OutputSignals=Body.BdyFrm.Cg.Vel.xdot,Body.InertFrm.Cg.Disp.X,Body.InertFrm.Cg.Disp.Y,Body.InertFrm.Cg.Ang.psi,Body.BdyFrm.Cg.AngVel.r
  Bus Selector2 : BusSelector  OutputSignals=Err.LatErr.Err
  Constant1 : Constant  Value=origin(1)
  Constant2 : Constant  Value=origin(2)
  Constant3 : Constant  Value=origin(1)
  Constant4 : Constant  Value=origin(2)
  Demux : Demux  Outputs=3
  Demux1 : Demux  Outputs=3
  Gain : Gain
  Gain1 : Gain
  Ground : Ground
  Ground1 : Ground
  Integrator : Integrator
  MATLAB Function : MATLAB Function  TreatAsAtomicUnit=on
  MATLAB Function1 : MATLAB Function  TreatAsAtomicUnit=on
  Memory : Memory
  Mux : Mux  Inputs=3
  Mux1 : Mux  Inputs=3
  Mux2 : Mux  Inputs=2
  Mux4 : Mux  Inputs=3
  Mux5 : Mux  Inputs=2
  Mux6 : Mux  Inputs=2
  Predictive Driver1 : vehdynlibdriver/Predictive Driver  extAccelOvr=off  extDecelOvr=off  extAccelHld=off  extDecelHld=off  extAccelZero=off  extDecelZero=off  extSteerOvr=on  extSteerHld=off  extSteerZero=off  cntrlType=Predictive  cntrlTypeLat=Stanley  shftType=Reverse, Neutral, Drive  coordMode=SAE J670 (Z-down)  refType=Reference pose  velUnits=m/s  angUnits=rad  gearOut=on  steerOut=on  Kp=10  Ki=5  Kff=.1  Kg=0  VehVelVec=[0 100]  KffVec=[.1 .1]  KpVec=[10 10]  KiVec=[5 5]  KgVec=[0 0]  vnom=5  Kaw=1  tauerr=.01  tau=0.15  L=50  Kpt=15000  aR=200  bR=2.5  cR=.5  g=9.81  vecPose=on  dynamMode=on  PositionGainF=2.5  PositionGainR=2.5  YawRateGain=.2  DelayGain=.2  enableDrift=off  BetaRef=20*pi/180  KpBeta=1  KpDrift=2  KdDrift=1  KpPsi=6  KOmega=30  tOmega=1  a=VEH.FrontAxlePositionfromCG  b=VEH.RearAxlePositionfromCG  m=VEH.Mass  Cy_f=5000  Cy_r=70933  I=4013  Ksteer=18  theta=45*pi/180  Idl=3  Re=.3  lambda_mu=1  GearInit=0  tShift=.1  pdlVec=[0.1 0.4 0.5 0.9]  upShftTbl=[-1 12.9375 26.4375 39.9375 51.18749999999999 62.4375 72.84375 83.25;-1 16.3125 29.8125 43.3125 54.5624 65.8125 76.78125 87.75;-1 19.6875 33.1875 46.68749999999999 57.9375 69.1875 80.71875 92.25;-1 33 52.5 77.25 100.5 138.75 161.875 185]  dwnShftTbl=[-1 12.9375 26.4375 39.9375 51.18749999999999 62.4375 72.84375 83.25;-1 16.3125 29.8125 43.3125 54.5624 65.8125 76.78125 87.75;-1 19.6875 33.1875 46.68749999999999 57.9375 69.1875 80.71875 92.25;-1 33 52.5 77.25 100.5 138.75 161.875 185]  tClutch=.5  tRev=.5  tPark=120  UpGearVec="[0  1  2  3  4  5  6  7]"  DownGearVec="[1  2  3  4  5  6  7  8]"  aMode=2
  Reshape1 : Reshape  OutputDimensionality=Row vector (2-D)  OutputDimensions=[1,3]
  Reshape2 : Reshape  OutputDimensionality=Row vector (2-D)
  Signal Specification : SignalSpecification  Unit=m
  Signal Specification3 : SignalSpecification  Unit=m/s
  Stop Simulation : Stop
  Subsystem : Subsystem
  Terminator{,1..7} (8 alike) : Terminator
  Traveling distance : simulink/Logic and Bit Operations/Compare To Constant  relop=>=  const=totalDistance*2  OutDataTypeStr=boolean  ZeroCross=off
  Unit Conversion1 : UnitConversion
  Unit Conversion3 : UnitConversion
  Out1 : Outport
  tag scope: RefXY=global
  wires:
  Predictive Driver1/5 -> Bus Creator/4  "GearCmd"
  Bus Selector/4 -> Mux2/1  "<Xdot>"
  Predictive Driver1/1 -> Terminator/1, Bus Selector2/1
  Reshape1/1 -> Predictive Driver1/8  "currentPose"
  Ground/1 -> Predictive Driver1/5
  Predictive Driver1/2 -> Memory/1  "SteerCmd"
  Bus Selector/2 -> Mux1/2, Gain/1  "<Y>"
  Mux2/1 -> Terminator1/1
  Traveling distance/1 -> Stop Simulation/1
  Integrator/1 -> Signal Specification/1
  Bus Selector/6 -> Gain1/1, Integrator/1  "<xdot>"
  Bus Selector1/4 -> Mux4/3  "<psi>"
  Bus Selector/5 -> Mux2/2  "<Ydot>"
  Bus Creator/1 -> Out1/1
  Predictive Driver1/3 -> Bus Creator/2  "AccelCmd"
  Bus Selector1/2 -> Mux4/1  "<X>"
  Bus Selector1/1 -> Unit Conversion1/1  "<xdot>"
  Predictive Driver1/4 -> Bus Creator/3  "DecelCmd"
  Bus Selector/3 -> Mux1/3  "<psi>"
  Bus Selector/1 -> Mux1/1  "<X>"
  Bus Selector1/3 -> Mux4/2  "<Y>"
  Unit Conversion1/1 -> Predictive Driver1/7
  Signal Specification/1 -> [Mileage]  "Mileage"
  1-D Lookup Table1/1 -> Signal Specification3/1  "LngRef"
  Signal Specification3/1 -> Unit Conversion3/1
  Unit Conversion3/1 -> Predictive Driver1/1
  In1/1 -> Bus Selector/1, Bus Selector1/1
  [Mileage] -> Traveling distance/1
  [Mileage] -> Subsystem/1(In1), 1-D Lookup Table4/1, 1-D Lookup Table3/1, 1-D Lookup Table1/1, 1-D Lookup Table2/1
  [RefXY] -> Demux/1  "RefPosition"
  Mux4/1 -> Reshape1/1
  Memory/1 -> Bus Creator/1  "SteerCmd"
  1-D Lookup Table2/1 -> Mux/1
  1-D Lookup Table3/1 -> Mux/2
  1-D Lookup Table4/1 -> Mux/3
  Mux/1 -> Reshape2/1  "PoseRef2"
  Reshape2/1 -> [RefXY], Predictive Driver1/2  "PoseRef2"
  Mux1/1 -> Demux1/1  "VehiclePosition"
  MATLAB Function/1(lat) -> Mux5/1
  Demux/1 -> MATLAB Function/1(x)
  Demux/2 -> MATLAB Function/2(y)
  Constant1/1 -> MATLAB Function/3(lat0)
  Constant2/1 -> MATLAB Function/4(lon0)
  Mux5/1 -> Terminator2/1  "RefLatLon"
  MATLAB Function/2(lon) -> Mux5/2
  Demux1/1 -> MATLAB Function1/1(x)
  Demux1/2 -> MATLAB Function1/2(y)
  MATLAB Function1/2(lon) -> Mux6/2
  Mux6/1 -> [GPS]  "VehLatLon"
  MATLAB Function1/1(lat) -> Mux6/1
  Constant3/1 -> MATLAB Function1/3(lat0)
  Constant4/1 -> MATLAB Function1/4(lon0)
  Bus Selector1/5 -> Predictive Driver1/9  "<r>"
  [GPS] -> Bus Creator/5  "GPS"
  Bus Selector2/1 -> Terminator3/1  "<Err>"
  Subsystem/2(Out2) -> Predictive Driver1/4
  Subsystem/1(Out1) -> Predictive Driver1/3
  Ground1/1 -> Predictive Driver1/6
  Demux/3 -> Terminator4/1
  Demux1/3 -> Terminator5/1
  Gain/1 -> Terminator6/1  "vert_turn"
  Gain1/1 -> Terminator7/1  "veh_velocity"

== system PassCarModel_RL_config/Vehicle with driver and environment/Environment ==
  In Bus Element2 : Inport  PortName=VehFdbk
  In Bus Element8 : Inport  PortName=VehFdbk  Element=Body.InertFrm
  In Bus Element9 : Inport  PortName=VehFdbk  Element=Body.InertFrm
  In Bus Element1 : Inport  PortName=VehFdbk  Element=Body.InertFrm.Cg.Disp
  Bus Creator2 : BusCreator  Inputs=2
  Bus Selector : BusSelector  OutputSignals=FrntAxl.Lft.Disp.X,FrntAxl.Rght.Disp.X,RearAxl.Lft.Disp.X,RearAxl.Rght.Disp.X
  Bus Selector1 : BusSelector  OutputSignals=FrntAxl.Lft.Disp.Y,FrntAxl.Rght.Disp.Y,RearAxl.Lft.Disp.Y,RearAxl.Rght.Disp.Y
  Constant1 : Constant  Value=0
  Constant2 : Constant  Value=0
  Constant6 : Constant  Value=0
  Ground Feedback : Subsystem  Variant=on  VariantControlMode=label  LabelModeActiveChoice=0
  Road Track Friction : Subsystem  mask(Road Track Friction){surface_popup=Constant friction coefficient scaling factor, lambda_g=.6, lambda_r=.4, r_x0=175, r_y0=-100, r_xw=1000, r_yw=500, aMode=2}
      mask prompts: surface_popup "vdynblks:vehdynManFriction:blkPrm_surface_popup"; lambda_g "vdynblks:vehdynManFriction:blkPrm_lambda_g"; lambda_r "vdynblks:vehdynManFriction:blkPrm_lambda_r"; r_x0 "vdynblks:vehdynManFriction:blkPrm_r_x0"; r_y0 "vdynblks:vehdynManFriction:blkPrm_r_y0"; r_xw "vdynblks:vehdynManFriction:blkPrm_r_xw"; r_yw "vdynblks:vehdynManFriction:blkPrm_r_yw"
      mask init:
      | % Scaling factor for the friction coefficient around the rectangular region
      | mutable = [lambda_g, lambda_g, lambda_g, lambda_g;
      |            lambda_g, lambda_r, lambda_r, lambda_g; 
      |            lambda_g, lambda_r, lambda_r, lambda_g; 
      |            lambda_g, lambda_g, lambda_g, lambda_g ];
      |        
      | 
      | % The step is distance between breakpoint near the boundary of high and
      | % low friction coefficient
      | 
      | step = 0.01 ; 
      | 
      | % In the mask initialization, xbr and ybr breakpoints are with respect to
      | % Body fixed coordinate system. At time t=0, xbr and ybr breakpoints
      | % updates to Earth (Inertial) Fixed coordinate system. The breakpoints for
      | % the lookup table are added via inputs.
      | 
      | xbr = [(r_x0 - step) , (r_x0 + step), (r_x0 + r_xw - step) , (r_x0 + r_xw + step) ];
      | ybr = [(r_y0 - step) , (r_y0 + step), (r_y0 + r_yw - step) , (r_y0 + r_yw + step) ];
      | 
      | 
      | % To check if the created track is split mu or constant mu
      | 
      | surface_popup = get_param(gcb, 'surface_popup');
      | 
      | if strcmp(surface_popup, 'Split friction coefficient scaling factor')
      |     SplitLambdaTrck = 1;
      | elseif strcmp(surface_popup, 'Constant friction coefficient scaling factor')
      |     SplitLambdaTrck = 0;
      | end
      mask Help: eval('vdynblkshelp(''vdynblkstrack'')');
      mask TypeOptions surface_popup: vdynblks:vehdynManFriction:blkCmb_surface_popup_c1 | vdynblks:vehdynManFriction:blkCmb_surface_popup_c2
      mask Callback surface_popup:
      | surface_popup = get_param(gcb, 'surface_popup');
      | m = Simulink.Mask.get(gcb);
      | 
      | lambda_g = m.getParameter('lambda_g');
      | lambda_r = m.getParameter('lambda_r');
      | r_x0 = m.getParameter('r_x0');
      | r_y0 = m.getParameter('r_y0');
      | r_xw = m.getParameter('r_xw');
      | r_yw = m.getParameter('r_yw');
      | %track_view = m.getParameter('track_view');
      | 
      | 
      | if strcmp(surface_popup, 'Split friction coefficient scaling factor')
      |     lambda_g.Visible = 'on';
      |     lambda_r.Visible = 'on';
      |     r_x0.Visible = 'on';
      |     r_y0.Visible = 'on';
      |     r_xw.Visible = 'on';
      |     r_yw.Visible = 'on';
      |     %track_view.Visible = 'on';
      | 
      | elseif strcmp(surface_popup,'Constant friction coefficient scaling factor')
      |     lambda_g.Visible = 'on';
      |     lambda_r.Visible = 'off';
      |     r_x0.Visible = 'off';
      |     r_y0.Visible = 'off';
      |     r_xw.Visible = 'off';
      |     r_yw.Visible = 'off';
      |     %track_view.Visible = 'off';
      | end
      | [~]=autosharedicon('autolibutils',gcb,0);
      mask DialogControl DescGroupVar Prompt: Road Track Friction
      mask DialogControl DescTextVar Prompt: vdynblks:vehdynManFriction:blkDesc
      mask DialogControl surface_popup Prompt: Type of surface:
      mask DialogControl lambda_g Prompt: Scaling factor for the friction coefficient of ground, lambda_g :
      mask DialogControl lambda_r Prompt: Scaling factor for the friction coefficient of rectangular surface, lambda_r :
      mask DialogControl r_x0 Prompt: X coordinate of lower left corner of rectangular surface, r_x0 [m]:
      mask DialogControl r_y0 Prompt: Y coordinate of lower left corner of rectangular surface, r_y0 [m]:
      mask DialogControl r_xw Prompt: Rectangular surface width in X direction, r_xw [m]:
      mask DialogControl r_yw Prompt: Rectangular surface width in Y direction, r_yw [m]:
  Vector Concatenate1 : Concatenate  NumInputs=3
  Wheel Coordinates : Subsystem
  Env : Outport  VectorParamsAs1DForOutWhenUnconnected=off
  wires:
  Bus Selector1/4 -> Wheel Coordinates/8(RearAxlRghtY)  "<Y>"
  Bus Selector1/3 -> Wheel Coordinates/7(RearAxlLftY)  "<Y>"
  In Bus Element9/1 -> Bus Selector1/1
  Bus Selector1/2 -> Wheel Coordinates/6(FrntAxlRghtY)  "<Y>"
  Bus Selector1/1 -> Wheel Coordinates/5(FrntAxlLftY)  "<Y>"
  In Bus Element8/1 -> Bus Selector/1
  Constant1/1 -> Vector Concatenate1/1  "X"
  Constant6/1 -> Vector Concatenate1/3  "Z"
  Bus Creator2/1 -> Env/1
  Constant2/1 -> Vector Concatenate1/2  "Y"
  Vector Concatenate1/1 -> Bus Creator2/1  "Wind"
  Ground Feedback/1(Ground) -> Bus Creator2/2  "Gnd"
  Road Track Friction/1(FricCoeffLambda) -> Ground Feedback/1(Friction)
  Wheel Coordinates/1(XWhl) -> Road Track Friction/1(XWhl)
  Wheel Coordinates/2(YWhl) -> Road Track Friction/2(YWhl)
  Bus Selector/1 -> Wheel Coordinates/1(FrntAxlLftX)  "<X>"
  Bus Selector/2 -> Wheel Coordinates/2(FrntAxlRghtX)  "<X>"
  Bus Selector/3 -> Wheel Coordinates/3(RearAxlLftX)  "<X>"
  Bus Selector/4 -> Wheel Coordinates/4(RearAxlRghtX)  "<X>"
  In Bus Element1/1 -> Road Track Friction/3(Cg)
  In Bus Element2/1 -> Ground Feedback/2(VehFdbk)

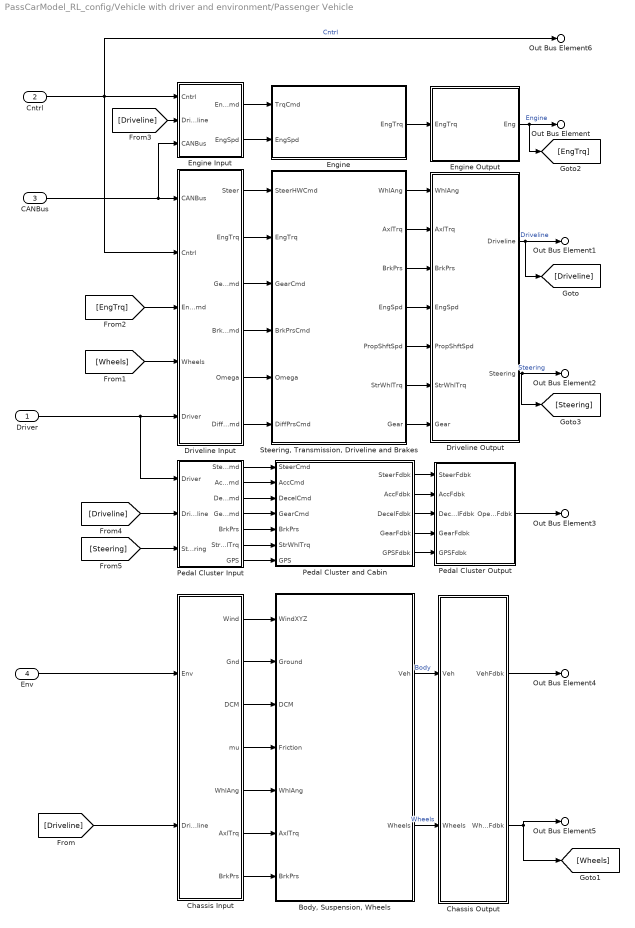
== system PassCarModel_RL_config/Vehicle with driver and environment/Passenger Vehicle ==
  Driver : Inport
  Cntrl : Inport  Port=2
  CANBus : Inport  Port=3
  Env : Inport  Port=4
  "Body, Suspension, Wheels" : Subsystem  Variant=on  VariantControlMode=label  LabelModeActiveChoice=3
  Chassis Input : Subsystem
  Chassis Output : Subsystem
  Driveline Input : Subsystem  mask{ControlMode=CAN}
      mask prompts: ControlMode "Select control mode"
      mask DialogControl DescTextVar Prompt: If CAN is selected the control signals are received from the CAN bus.
  Driveline Output : Subsystem
  Engine : Subsystem  Variant=on  VariantControlMode=label  LabelModeActiveChoice=0
  Engine Input : Subsystem  mask{ControlMode=CAN}
      mask prompts: ControlMode "Select control mode"
      mask DialogControl DescTextVar Prompt: If CAN is selected the control signals are received from the CAN bus.
  Engine Output : Subsystem
  Pedal Cluster Input : Subsystem
  Pedal Cluster Output : Subsystem
  Pedal Cluster and Cabin : Subsystem
  "Steering, Transmission, Driveline and Brakes" : Subsystem  Variant=on  VariantControlMode=label  LabelModeActiveChoice=0
  Out Bus Element : Outport  PortName=VehFdbk  Element=Engine
  Out Bus Element3 : Outport  PortName=VehFdbk  Element=Driver
  Out Bus Element4 : Outport  PortName=VehFdbk  Element=Body
  Out Bus Element5 : Outport  PortName=VehFdbk  Element=Wheels
  Out Bus Element1 : Outport  PortName=VehFdbk  Element=Driveline
  Out Bus Element2 : Outport  PortName=VehFdbk  Element=Steering
  Out Bus Element6 : Outport  PortName=VehFdbk  Element=Cntrl
  wires:
  Env/1 -> Chassis Input/1(Env)
  Chassis Input/1(Wind) -> "Body, Suspension, Wheels"/1(WindXYZ)
  "Steering, Transmission, Driveline and Brakes"/1(WhlAng) -> Driveline Output/1(WhlAng)
  "Steering, Transmission, Driveline and Brakes"/2(AxlTrq) -> Driveline Output/2(AxlTrq)
  "Steering, Transmission, Driveline and Brakes"/3(BrkPrs) -> Driveline Output/3(BrkPrs)
  "Steering, Transmission, Driveline and Brakes"/4(EngSpd) -> Driveline Output/4(EngSpd)
  "Steering, Transmission, Driveline and Brakes"/5(PropShftSpd) -> Driveline Output/5(PropShftSpd)
  Driver/1 -> Pedal Cluster Input/1(Driver), Driveline Input/5(Driver)
  Cntrl/1 -> Driveline Input/2(Cntrl), Out Bus Element6/1, Engine Input/1(Cntrl)  "Cntrl"
  Driveline Input/1(Steer) -> "Steering, Transmission, Driveline and Brakes"/1(SteerHWCmd)
  Driveline Input/3(GearCmd) -> "Steering, Transmission, Driveline and Brakes"/3(GearCmd)
  Driveline Input/4(BrkPrsCmd) -> "Steering, Transmission, Driveline and Brakes"/4(BrkPrsCmd)
  Driveline Input/5(Omega) -> "Steering, Transmission, Driveline and Brakes"/5(Omega)
  Engine/1(EngTrq) -> Engine Output/1("EngTrq ")
  Engine Input/1(EngTrqCmd) -> Engine/1(TrqCmd)
  Engine Input/2(EngSpd) -> Engine/2(EngSpd)
  Engine Output/1(Eng) -> Out Bus Element/1, [EngTrq]  "Engine"
  [Wheels] -> Driveline Input/4(Wheels)
  [EngTrq] -> Driveline Input/3(EngTrqCmd)
  [Driveline] -> Engine Input/2(Driveline)
  Driveline Input/6(DiffPrsCmd) -> "Steering, Transmission, Driveline and Brakes"/6(DiffPrsCmd)
  "Steering, Transmission, Driveline and Brakes"/6(StrWhlTrq) -> Driveline Output/6(StrWhlTrq)
  Pedal Cluster Output/1(OperatorFdbk) -> Out Bus Element3/1
  Pedal Cluster and Cabin/1(SteerFdbk) -> Pedal Cluster Output/1(SteerFdbk)
  Pedal Cluster and Cabin/2(AccFdbk) -> Pedal Cluster Output/2(AccFdbk)
  Pedal Cluster and Cabin/3(DecelFdbk) -> Pedal Cluster Output/3(DecelFdbk)
  Pedal Cluster and Cabin/4(GearFdbk) -> Pedal Cluster Output/4(GearFdbk)
  Pedal Cluster Input/4(GearCmd) -> Pedal Cluster and Cabin/4(GearCmd)
  Pedal Cluster Input/3(DecelCmd) -> Pedal Cluster and Cabin/3(DecelCmd)
  Pedal Cluster Input/2(AccelCmd) -> Pedal Cluster and Cabin/2(AccCmd)
  Pedal Cluster Input/1(SteerCmd) -> Pedal Cluster and Cabin/1(SteerCmd)
  [Driveline] -> Pedal Cluster Input/2(Driveline)
  Pedal Cluster Input/5(BrkPrs) -> Pedal Cluster and Cabin/5(BrkPrs)
  [Steering] -> Pedal Cluster Input/3(Steering)
  Pedal Cluster Input/6(StrWhlTrq) -> Pedal Cluster and Cabin/6(StrWhlTrq)
  Chassis Output/2(WheelsFdbk) -> Out Bus Element5/1, [Wheels]
  Chassis Output/1(VehFdbk) -> Out Bus Element4/1
  "Steering, Transmission, Driveline and Brakes"/7(Gear) -> Driveline Output/7(Gear)
  Driveline Output/1(Driveline) -> Out Bus Element1/1, [Driveline]  "Driveline"
  Driveline Output/2(Steering) -> [Steering], Out Bus Element2/1  "Steering"
  Chassis Input/3(DCM) -> "Body, Suspension, Wheels"/3(DCM)
  Chassis Input/6(AxlTrq) -> "Body, Suspension, Wheels"/6(AxlTrq)
  "Body, Suspension, Wheels"/1(Veh) -> Chassis Output/1(Veh)  "Body"
  "Body, Suspension, Wheels"/2(Wheels) -> Chassis Output/2(Wheels)  "Wheels"
  Chassis Input/7(BrkPrs) -> "Body, Suspension, Wheels"/7(BrkPrs)
  Chassis Input/2(Gnd) -> "Body, Suspension, Wheels"/2(Ground)
  Chassis Input/5(WhlAng) -> "Body, Suspension, Wheels"/5(WhlAng)
  Chassis Input/4(mu) -> "Body, Suspension, Wheels"/4(Friction)
  [Driveline] -> Chassis Input/2(Driveline)
  CANBus/1 -> Engine Input/3(CANBus), Driveline Input/1(CANBus)
  Driveline Input/2(EngTrq) -> "Steering, Transmission, Driveline and Brakes"/2(EngTrq)
  Pedal Cluster and Cabin/5(GPSFdbk) -> Pedal Cluster Output/5(GPSFdbk)
  Pedal Cluster Input/7(GPS) -> Pedal Cluster and Cabin/7(GPS)

== system PassCarModel_RL_config/Vehicle with driver and environment/Sensors ==
  VehFdbk : Inport
  Env : Inport  Port=2
  Bus Creator1 : BusCreator  Inputs=2
  Bus Selector : BusSelector  OutputSignals=Body.BdyFrm.Cg.Acc.ax,Body.BdyFrm.Cg.Acc.ay,Body.BdyFrm.Cg.Acc.az  OutputAsBus=on
  Bus Selector1 : BusSelector  OutputSignals=Body.BdyFrm.Cg.AngVel.p,Body.BdyFrm.Cg.AngVel.q,Body.BdyFrm.Cg.AngVel.r  OutputAsBus=on
  Bus Selector2 : BusSelector  OutputSignals=Body.BdyFrm.Cg.AngAcc.pdot,Body.BdyFrm.Cg.AngAcc.qdot,Body.BdyFrm.Cg.AngAcc.rdot  OutputAsBus=on
  Bus Selector3 : BusSelector  OutputSignals=Driver  OutputAsBus=on
  Bus Selector4 : BusSelector  OutputSignals=Engine.EngTrq,Driveline.EngSpd  OutputAsBus=on
  Bus Selector5 : BusSelector  OutputSignals=Driveline.BrkPrs,Wheels.TireFrame.Kappa,Wheels.TireFrame.Alpha,Wheels.TireFrame.Omega  OutputAsBus=on
  Bus Selector6 : BusSelector  OutputSignals=Driveline.PropShftSpd,Driveline.AxlTrq  OutputAsBus=on
  Bus to Vector : BusToVector
  Bus to Vector1 : BusToVector
  Bus to Vector2 : BusToVector
  Constant : Constant  Value=[0,0,0]
  Constant1 : Constant  Value=[0,0,9.81]
  Three-axis Inertial Measurement Unit : vehdynlibsens/Three-axis Inertial Measurement Unit  units=Metric (MKS)  imu=[0 0 0]  i_Ts=0  dtype_a=off  w_a=190  z_a=0.707  a_sf_cc=[1 0 0; 0 1 0; 0 0 1]  a_bias=[0 0 0]  a_sat="[-inf  -inf  -inf  inf inf inf]"  dtype_g=off  w_g=190  z_g=0.707  g_sf_cc=[1 0 0; 0 1 0; 0 0 1]  g_bias=[0 0 0]  g_sens=[0 0 0]  g_sat="[-inf  -inf  -inf  inf inf inf]"  i_rand=on  i_seeds=[23093 23094 23095 23096 23097 23098]  i_pow=[0.001 0.001 0.001 0.0001 0.0001 0.0001]  aMode=2
  Unit Conversion : UnitConversion
  Out Bus Element : Outport  PortName=CntrlRx  Element=Driver
  Out Bus Element1 : Outport  PortName=CntrlRx  Element=Engine
  Out Bus Element2 : Outport  PortName=CntrlRx  Element=Trans
  Out Bus Element3 : Outport  PortName=CntrlRx  Element=Wheels
  Out Bus Element4 : Outport  PortName=CntrlRx  Element=IMU
  Out Bus Element5 : Outport  PortName=CntrlRx  Element=Env
  wires:
  VehFdbk/1 -> Bus Selector/1, Bus Selector2/1, Bus Selector1/1, Bus Selector6/1, Bus Selector3/1, Bus Selector4/1, Bus Selector5/1  "VehFdbk"
  Bus Creator1/1 -> Out Bus Element4/1
  Three-axis Inertial Measurement Unit/1 -> Bus Creator1/1  "Acc"
  Three-axis Inertial Measurement Unit/2 -> Bus Creator1/2  "pqr"
  Bus Selector/1 -> Bus to Vector/1
  Bus to Vector/1 -> Unit Conversion/1
  Bus Selector1/1 -> Bus to Vector1/1
  Bus to Vector1/1 -> Three-axis Inertial Measurement Unit/2
  Env/1 -> Out Bus Element5/1
  Bus Selector2/1 -> Bus to Vector2/1
  Bus to Vector2/1 -> Three-axis Inertial Measurement Unit/3
  Constant/1 -> Three-axis Inertial Measurement Unit/4
  Constant1/1 -> Three-axis Inertial Measurement Unit/5
  Unit Conversion/1 -> Three-axis Inertial Measurement Unit/1
  Bus Selector3/1 -> Out Bus Element/1
  Bus Selector4/1 -> Out Bus Element1/1
  Bus Selector5/1 -> Out Bus Element3/1
  Bus Selector6/1 -> Out Bus Element2/1
